simulink model "modelo_EAF"  (R2017b)
settings: Solver=ode8  StartTime=0.0  StopTime=time_sim  FixedStep=1/Fs  MaxStep=50e-6  RelTol=1e-3
values from neighbouring files (symbols this model uses):
  beta = Y(n,5)    [datos_entrenamiento.m]    (also in hiperparametros.m = ypred(5); prediccion.m = round(beta*100,2); sensibilidad.m = ypred(5))
  Fs = 4*Fm; save([PathFolder '/Fs'],'Fs')    [datos_entrenamiento.m]    (also in prediccion.m = 4*Fm; sensibilidad.m = 4*Fm)
  k1 = Y(n,1)    [datos_entrenamiento.m]    (also in hiperparametros.m = ypred(1); prediccion.m = round(k1*10000,2); sensibilidad.m = ypred(1))
  k2 = Y(n,2)    [datos_entrenamiento.m]    (also in hiperparametros.m = ypred(2); prediccion.m = round(k2*10,2); sensibilidad.m = ypred(2))
  k3 = Y(n,3)    [datos_entrenamiento.m]    (also in hiperparametros.m = ypred(3); prediccion.m = round(k3*15,2); sensibilidad.m = ypred(3))
  Lc = Y(n,8)    [datos_entrenamiento.m]    (also in hiperparametros.m = ypred(8); prediccion.m = Lc*0.00001; sensibilidad.m = ypred(8))
  Rc = Y(n,7)    [datos_entrenamiento.m]    (also in hiperparametros.m = ypred(7); prediccion.m = Rc*0.001; sensibilidad.m = ypred(7))
  s = Y(n,4)    [datos_entrenamiento.m]    (also in hiperparametros.m = ypred(4); prediccion.m = round(s*100,2); sensibilidad.m = ypred(4))
  w = Y(n,6)    [datos_entrenamiento.m]    (also in hiperparametros.m = ypred(6); prediccion.m = round(w*1,2); sensibilidad.m = ypred(6))
libraries: powerlib x1
settings Model: Creator=Administrador  LastModifiedBy=Jesser
settings DataIOCC: SaveFormat=Array  SignalLoggingSaveFormat=ModelDataLogs  SaveOutput=off  TimeSaveName=t
settings OptimizationCC: ExpressionDepthLimit=2147483647  InitFltsAndDblsToZero=on  LifeSpan=inf
settings DebuggingCC: UnderspecifiedInitializationDetection=Classic  MergeDetectMultiDrivingBlocksExec=none  SolverPrmCheckMsg=warning  FcnCallInpInsideContextMsg=warning  UnconnectedInputMsg=none  UnconnectedOutputMsg=none  UnconnectedLineMsg=none  StateNameClashWarn=warning  SFUnexpectedBacktrackingDiag=warning  SFNoUnconditionalDefaultTransitionDiag=warning  SFExecutionAtInitializationDiag=none
settings HardwareCC: ProdBitPerPointer=32  ProdBitPerSizeT=32  ProdBitPerPtrDiffT=32  ProdLargestAtomicFloat=None  ProdIntDivRoundTo=Undefined  ProdEndianess=Unspecified  ProdWordSize=32  ProdHWDeviceType=32-bit Generic
settings ModelReferenceCC: PropagateSignalLabelsOutOfModel=off
settings CodeAppCC: StateflowObjectComments=on
settings GRTTargetCC: TargetLangStandard=C89/C90 (ANSI)  GeneratePreprocessorConditionals=Disable all  CombineOutputUpdateFcns=off  GRTInterface=on
settings ConfigComp: CovMetricSettings=dw  CovHtmlReporting=on  CovSaveCumulativeToWorkspaceVar=on  CovSaveSingleToWorkspaceVar=on  CovExternalEMLEnable=off
settings SimscapeCC: SimscapeNormalizeSystem=off

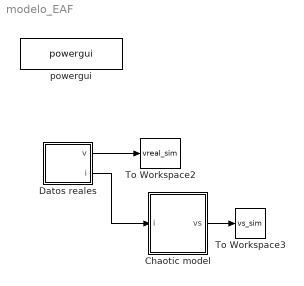
== system modelo_EAF ==
  Chaotic model : Subsystem
  Datos reales : Subsystem
  To Workspace2 : ToWorkspace  VariableName=vreal_sim  SampleTime=-1
  To Workspace3 : ToWorkspace  VariableName=vs_sim  SampleTime=-1
  powergui : powerlib/powergui  SimulationMode=Discrete  SampleTime=1/Fs  frequency=60  Iterations=50  frequencyindice=0  Pbase=100e6  ErrMax=1e-4  UnitsV=kV  UnitsW=MW  buscounter=0  FunctionMessages=off  echomessages=off  EnableUseOfTLC=off  CurrentSourceSwitches=off  DisableSnubberDevices=off  DisableRonSwitches=off  DisableVfSwitches=off  DisplayEquations=off  SolverType=Tustin/Backward Euler (TBE)  Interpol=off  ExternalGateDelay=off  methode=off  Ts=100  x0status=blocks  SPID=off  SwTol=0  HookPort=off  RestoreLinks=warning  ResistiveCurrentMeasurement=off  Frange=[0:2:500]  Ylog=off  Xlog=on  ShowGrid=off  save=off  variable=ZData  structure=0  ZoomFFT=on  StartTime=0.0  cycles=1  DisplayStyle=1  fundamental=60  FreqAxis=off  MaxFrequency=1000  frequencyindicesteady=1  RmsSteady=1  display=off
  wires:
  Datos reales/1(v) -> To Workspace2/1
  Datos reales/2(i) -> Chaotic model/1(i)
  Chaotic model/1(vs) -> To Workspace3/1

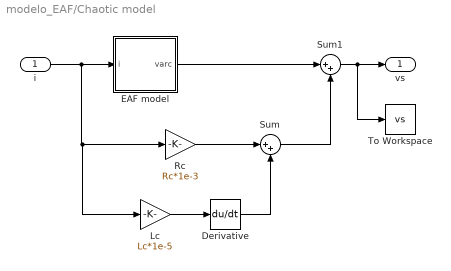
== system modelo_EAF/Chaotic model ==
  i : Inport
  Derivative : Derivative
  EAF model : Subsystem
  Lc : Gain  Gain=Lc*1e-5
  Rc : Gain  Gain=Rc*1e-3
  Sum : Sum  Inputs=|++
  Sum1 : Sum  Inputs=|++
  To Workspace : ToWorkspace  VariableName=vs  SampleTime=-1
  vs : Outport
  wires:
  EAF model/1(varc) -> Sum1/1
  i/1 -> Lc/1, Rc/1, EAF model/1(i)
  Rc/1 -> Sum/1
  Sum/1 -> Sum1/2
  Sum1/1 -> To Workspace/1, vs/1
  Derivative/1 -> Sum/2
  Lc/1 -> Derivative/1

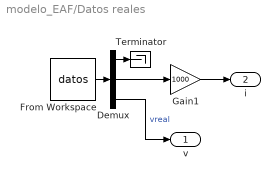
== system modelo_EAF/Datos reales ==
  Demux : Demux  Outputs=3
  From Workspace : FromWorkspace  VariableName=datos  SampleTime=0
  Gain1 : Gain  Gain=1000
  Terminator : Terminator
  v : Outport
  i : Outport  Port=2
  wires:
  From Workspace/1 -> Demux/1
  Demux/1 -> Terminator/1
  Demux/3 -> v/1  "vreal"
  Demux/2 -> Gain1/1
  Gain1/1 -> i/1

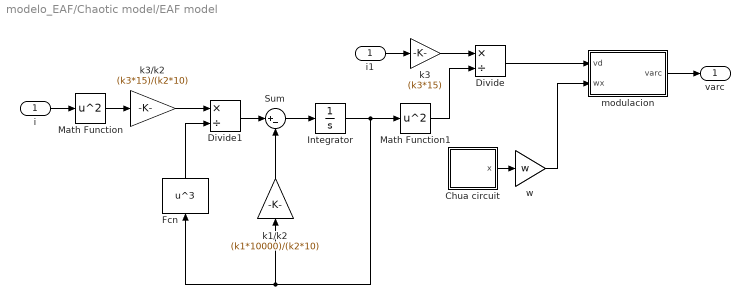
== system modelo_EAF/Chaotic model/EAF model ==
  i : Inport
  "Chua circuit " : Subsystem
  Divide : Product  Inputs=*/
  Divide1 : Product  Inputs=*/
  Fcn : Fcn  Expr=u^3
  Integrator : Integrator  InitialCondition=1e-0
  Math Function : Math  Operator=square  SaturateOnIntegerOverflow=on
  Math Function1 : Math  Operator=square  SaturateOnIntegerOverflow=on
  Sum : Sum  Inputs=|+-
  i1 : InportShadow
  k1/k2 : Gain  Gain=(k1*10000)/(k2*10)
  k3 : Gain  Gain=(k3*15)
  k3/k2 : Gain  Gain=(k3*15)/(k2*10)
  modulacion : Subsystem
  w : Gain  Gain=w
  varc : Outport
  wires:
  Math Function/1 -> k3/k2/1
  Fcn/1 -> Divide1/2
  Divide1/1 -> Sum/1
  k1/k2/1 -> Sum/2
  Sum/1 -> Integrator/1
  k3/k2/1 -> Divide1/1
  k3/1 -> Divide/1
  Math Function1/1 -> Divide/2
  i/1 -> Math Function/1
  i1/1 -> k3/1
  Integrator/1 -> Math Function1/1, Fcn/1, k1/k2/1
  Divide/1 -> modulacion/1(vd)
  modulacion/1(varc) -> varc/1
  "Chua circuit "/1(x) -> w/1
  w/1 -> modulacion/2(wx)

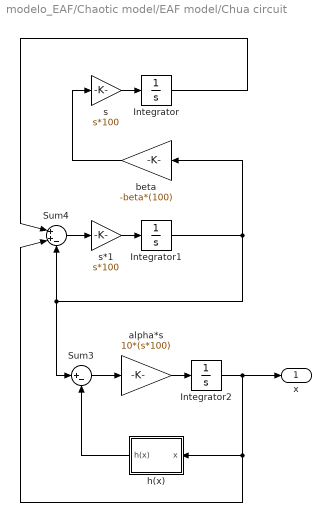
== system modelo_EAF/Chaotic model/EAF model/Chua circuit  ==
  Integrator : Integrator
  Integrator1 : Integrator
  Integrator2 : Integrator  InitialCondition=1
  Sum3 : Sum  Inputs=|+-
  Sum4 : Sum  Inputs=|++-
  alpha*s : Gain  Gain=10*(s*100)
  beta : Gain  Gain=-beta*(100)
  h(x) : Subsystem
  s : Gain  Gain=s*100
  s*1 : Gain  Gain=s*100
  x : Outport
  wires:
  Integrator2/1 -> Sum4/2, h(x)/1(x), x/1
  h(x)/1(h(x)) -> Sum3/2
  Integrator/1 -> Sum4/1
  Integrator1/1 -> Sum3/1, Sum4/3, beta/1
  alpha*s/1 -> Integrator2/1
  Sum3/1 -> alpha*s/1
  beta/1 -> s/1
  s/1 -> Integrator/1
  Sum4/1 -> s*1/1
  s*1/1 -> Integrator1/1

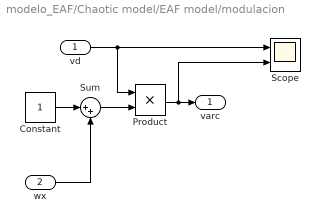
== system modelo_EAF/Chaotic model/EAF model/modulacion ==
  vd : Inport
  wx : Inport  Port=2
  Constant : Constant
  Product : Product
  Scope : Scope  NumInputPorts=2
  Sum : Sum  Inputs=|++
  varc : Outport
  wires:
  wx/1 -> Sum/2
  Constant/1 -> Sum/1
  Product/1 -> Scope/2, varc/1
  vd/1 -> Scope/1, Product/1
  Sum/1 -> Product/2

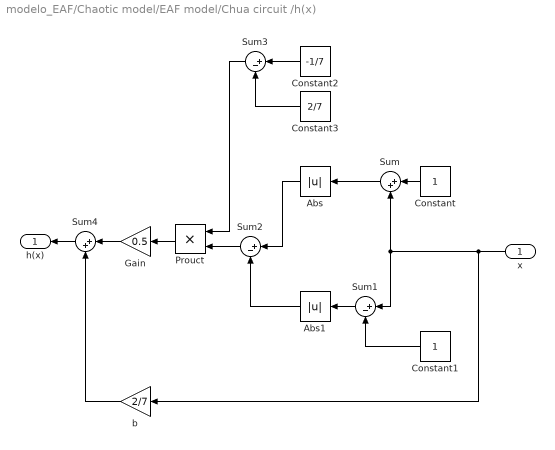
== system modelo_EAF/Chaotic model/EAF model/Chua circuit /h(x) ==
  x : Inport
  Abs : Abs
  Abs1 : Abs
  Constant : Constant
  Constant1 : Constant
  Constant2 : Constant  Value=-1/7
  Constant3 : Constant  Value=2/7
  Gain : Gain  Gain=0.5
  Prouct : Product  RndMeth=Zero
  Sum : Sum  Inputs=|++
  Sum1 : Sum  Inputs=|+-
  Sum2 : Sum  Inputs=|+-
  Sum3 : Sum  Inputs=|+-
  Sum4 : Sum  Inputs=|++
  b : Gain  Gain=2/7
  h(x) : Outport
  wires:
  x/1 -> Sum/2, Sum1/1, b/1
  Constant/1 -> Sum/1
  Constant1/1 -> Sum1/2
  Sum/1 -> Abs/1
  Sum1/1 -> Abs1/1
  Abs/1 -> Sum2/1
  Abs1/1 -> Sum2/2
  Sum2/1 -> Prouct/2
  Constant2/1 -> Sum3/1
  Constant3/1 -> Sum3/2
  Sum3/1 -> Prouct/1
  Prouct/1 -> Gain/1
  Gain/1 -> Sum4/1
  b/1 -> Sum4/2
  Sum4/1 -> h(x)/1
